simulink model "gm_sampleModel61753_pp_45_1_sub"  (R2023b)
settings: Solver=VariableStepAuto  StartTime=0.0  StopTime=10.0  RelTol=1e-3
libraries: simulink x43
(part 1 of 2)
settings Model: Creator=CW  LastModifiedBy=CW
settings OptimizationCC: BlockReduction=off  ConditionallyExecuteInputs=off
settings DebuggingCC: ArtificialAlgebraicLoopMsg=none  InheritedTsInSrcMsg=none

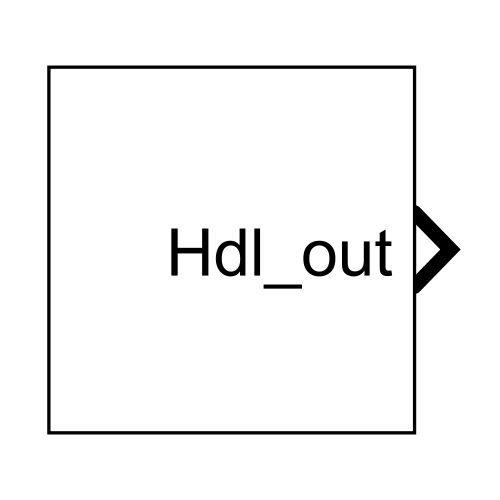
[thumbnail: Simulink's stored preview of the top-level diagram]
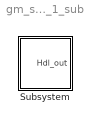
== system gm_sampleModel61753_pp_45_1_sub ==
  Subsystem : Subsystem

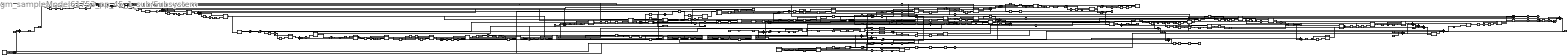
== system gm_sampleModel61753_pp_45_1_sub/Subsystem ==
  Reshape{,1..5} (6 alike) : Reshape
  cfblk1 : Subsystem
  cfblk{10,42,68,116,142,152} (6 alike) : Sum  OutDataTypeStr=uint8  AccumDataTypeStr=uint8  RndMeth=Nearest  SampleTime=1
  cfblk100 : Subsystem  mask(Real World Value Increment){}
      mask help: Simulink:masks:RealWorldValueIncrement_MD
      mask Display: disp('V++')
  cfblk101 : Subsystem
  cfblk{8,16,27,72,94,102,119..120,144,151} (10 alike) : Sum  Inputs=+  OutDataTypeStr=uint8
  cfblk{12,17,40,52,66,73,85,89,103,115,126} (11 alike) : Abs  SampleTime=1  OutDataTypeStr=uint8  SaturateOnIntegerOverflow=off
  cfblk{5,13,29,32,49,59,70,77,80..82,87,90,104,108,114,123,132,145} (19 alike) : Sum  OutDataTypeStr=uint8  AccumDataTypeStr=uint8  SampleTime=1
  cfblk{25..26,38,53,55,84,91,105,107} (9 alike) : MinMax  OutDataTypeStr=uint8
  cfblk{35,67,71,98,106,117} (6 alike) : Gain  Gain="fi(0,0,8,7,\"hex\",\"80\")"  ParamDataTypeStr=fixdt(0, 8, 7)  OutDataTypeStr=uint8  SampleTime=1
  cfblk109 : Subsystem
  cfblk10_const_val : Constant  Value=0  VectorParams1D=off  OutDataTypeStr=uint8  SampleTime=1
  cfblk{11,14,18,22,47,60,75,92,96,128,135} (11 alike) : Sum  Inputs=+-  OutDataTypeStr=uint8  AccumDataTypeStr=uint8  SampleTime=1
  cfblk{45,56,86,110,137,146..147} (7 alike) : Signum  SampleTime=1
  cfblk112 : Subsystem
  cfblk113 : Subsystem
  cfblk116_const_val : Constant  Value=0  VectorParams1D=off  OutDataTypeStr=uint8  SampleTime=1
  cfblk{15,23,28,34,36,118} (6 alike) : ComplexToRealImag  SampleTime=1
  cfblk121_inst : Subsystem
  cfblk124 : Subsystem
  cfblk125 : Subsystem
  cfblk127 : Subsystem
  cfblk129 : Subsystem
  cfblk130 : Subsystem  mask(Real World Value Increment){}
      mask help: Simulink:masks:RealWorldValueIncrement_MD
      mask Display: disp('V++')
  cfblk{39,44,61,78..79,99,131,136,149} (9 alike) : Product  Inputs=*/  OutDataTypeStr=uint8  RndMeth=Zero  SaturateOnIntegerOverflow=on  SampleTime=1
  cfblk133 : Subsystem
  cfblk134 : Subsystem
  cfblk138_inst : Subsystem
  cfblk139 : Subsystem  mask(Real World Value Increment){}
      mask help: Simulink:masks:RealWorldValueIncrement_MD
      mask Display: disp('V++')
  cfblk142_const_val : Constant  Value=0  VectorParams1D=off  OutDataTypeStr=uint8  SampleTime=1
  cfblk143 : Subsystem
  cfblk148 : Subsystem
  cfblk150 : Subsystem
  cfblk152_const_val : Constant  Value=0  VectorParams1D=off  OutDataTypeStr=uint8  SampleTime=1
  cfblk153 : Subsystem
  cfblk156 : Constant  OutDataTypeStr=uint8  SampleTime=1
  cfblk157 : Constant  OutDataTypeStr=uint8  SampleTime=1
  cfblk158 : Subsystem
  cfblk159 : Subsystem
  cfblk160 : Subsystem
  cfblk{161..164,166,168..171,173..178} (15 alike) : Delay  DelayLength=double(2)  InitialCondition=0  SampleTime=1
  cfblk165 : Subsystem
  cfblk167 : Subsystem
  cfblk172 : Subsystem
  cfblk{179,181..191,193} (13 alike) : DataTypeConversion  OutDataTypeStr=fixdt(0,8,0)
  cfblk180 : Subsystem
  cfblk19 : Subsystem
  cfblk192 : Subsystem
  cfblk194 : Subsystem
  cfblk2 : Subsystem  mask(Detect Rise Positive){vinit=double(0), InputProcessing=Elements as channels (sample based), OutDataTypeStr=uint8}
      mask prompts: vinit "Simulink:masks:InitialCondition_MP"; InputProcessing "Simulink:masks:InputProcessing_MP"; OutDataTypeStr "Simulink:masks:OutputDataType_MP"
      mask help: Simulink:masks:DetectRisePositive_MD
      mask init:
      | InputProcessing = 'Elements as channels (sample based)';
      | OutDataTypeStr = 'uint8';
      | vinit = double(0);
      mask TypeOptions InputProcessing: Simulink:masks:ColumnsAsChannelsFrameBased | Simulink:masks:ElementsAsChannelsSampleBased
      mask TypeOptions OutDataTypeStr: Simulink:masks:uint8 | Simulink:masks:boolean
      mask Display: fprintf('U > 0\n&  NOT\nU/z > 0')
  cfblk20 : Subsystem  mask(Real World Value Increment){}
      mask help: Simulink:masks:RealWorldValueIncrement_MD
      mask Display: disp('V++')
  cfblk21 : Subsystem
  cfblk24 : Subsystem
  cfblk28_term1 : Terminator
  cfblk3 : Subsystem  mask(Detect Rise Nonnegative){vinit=double(0), InputProcessing=Elements as channels (sample based), OutDataTypeStr=uint8}
      mask prompts: vinit "Simulink:masks:InitialCondition_MP"; InputProcessing "Simulink:masks:InputProcessing_MP"; OutDataTypeStr "Simulink:masks:OutputDataType_MP"
      mask help: Simulink:masks:DetectRiseNonnegative_MD
      mask init:
      | InputProcessing = 'Elements as channels (sample based)';
      | OutDataTypeStr = 'uint8';
      | vinit = double(0);
      mask TypeOptions InputProcessing: Simulink:masks:ColumnsAsChannelsFrameBased | Simulink:masks:ElementsAsChannelsSampleBased
      mask TypeOptions OutDataTypeStr: Simulink:masks:uint8 | Simulink:masks:boolean
      mask Display: fprintf('U >= 0\n&  NOT\nU/z >= 0')
  cfblk30 : Subsystem
  cfblk31_inst : Subsystem
  cfblk33 : Subsystem  mask(Real World Value Increment){}
      mask help: Simulink:masks:RealWorldValueIncrement_MD
      mask Display: disp('V++')
  cfblk37_inst : Subsystem
  cfblk4 : Subsystem  mask(Detect Fall Nonpositive){vinit=double(0), InputProcessing=Elements as channels (sample based), OutDataTypeStr=uint8}
      mask prompts: vinit "Simulink:masks:InitialCondition_MP"; InputProcessing "Simulink:masks:InputProcessing_MP"; OutDataTypeStr "Simulink:masks:OutputDataType_MP"
      mask help: Simulink:masks:DetectFallNonpositive_MD
      mask init:
      | InputProcessing = 'Elements as channels (sample based)';
      | OutDataTypeStr = 'uint8';
      | vinit = double(0);
      mask TypeOptions InputProcessing: Simulink:masks:ColumnsAsChannelsFrameBased | Simulink:masks:ElementsAsChannelsSampleBased
      mask TypeOptions OutDataTypeStr: Simulink:masks:uint8 | Simulink:masks:boolean
      mask Display: fprintf('U <= 0\n&  NOT\nU/z <= 0')
  cfblk41 : Subsystem
  cfblk42_const_val : Constant  Value=0  VectorParams1D=off  OutDataTypeStr=uint8  SampleTime=1
  cfblk43 : Subsystem
  cfblk46 : Subsystem
  cfblk48 : Subsystem
  cfblk50 : Subsystem
  cfblk51 : Subsystem
  cfblk54 : Subsystem
  cfblk57 : Subsystem
  cfblk58 : Subsystem
  cfblk62_inst : Subsystem
  cfblk65_inst : Subsystem
  cfblk68_const_val : Constant  Value=0  VectorParams1D=off  OutDataTypeStr=uint8  SampleTime=1
  cfblk69 : Subsystem
  cfblk6_inst : Subsystem
  cfblk7 : Subsystem
  cfblk74_inst : Subsystem
  cfblk76 : Subsystem
  cfblk83_inst : Subsystem
  cfblk88 : Subsystem
  cfblk9 : Subsystem
  cfblk93 : Subsystem
  cfblk95 : Subsystem
  cfblk97 : Subsystem
  compare{,1..2,4,6,11,14..16,20,22,24,26..28,33,36..38,41} (20 alike) : simulink/Logic and Bit Operations/Compare To Constant  relop=>=  const=0  OutDataTypeStr=boolean
  compare{5,7..10,12..13,17,19,21,23,25,29..30,32,34,39..40,42} (19 alike) : simulink/Logic and Bit Operations/Compare To Constant  relop=>=  const=255  OutDataTypeStr=boolean
  compare{3,18,31,35} (4 alike) : simulink/Logic and Bit Operations/Compare To Constant  relop=>=  const=1  OutDataTypeStr=boolean
  emi_{6,14,22,30,38,47,55,63,71,80,88,97,105,113,121,129,137,145,153,161,169,177,185,193,201,209,217,225,233,241,249,257,265,273,281,289,298,306,314,323,331,339,347} (43 alike) : DataTypeConversion  OutDataTypeStr=fixdt(0,8,0)
  emi_{7,15,23,31,56,64,89,106,114,122,146,186,210,218,250,266,282,299,307,348} (20 alike) : Delay  DelayLength=double(2)  InitialCondition=0  SampleTime=1
  emi_{48,130,234,332} (4 alike) : Delay  DelayLength=double(2)  InitialCondition=1  SampleTime=1
  emi_{39,72,81,98,138,154,162,170,178,194,202,226,242,258,274,290,315,324,340} (19 alike) : Delay  DelayLength=double(2)  InitialCondition=255  SampleTime=1
  Hdl_out : Outport  OutDataTypeStr=uint8  SampleTime=1
  wires:
  cfblk1/1(emi_2) -> cfblk60/1
  cfblk10/1 -> cfblk104/1
  cfblk100/1(y) -> cfblk189/1
  cfblk101/1(emi_18) -> cfblk25/1
  cfblk102/1 -> cfblk44/1, cfblk79/2
  cfblk103/1 -> cfblk147/1, cfblk100/1(u)
  cfblk104/1 -> cfblk176/1
  cfblk105/1 -> emi_130/1, cfblk148/1(emi_124), cfblk149/1
  cfblk106/1 -> cfblk47/2, cfblk146/1
  cfblk107/1 -> cfblk77/2, cfblk14/1
  cfblk108/1 -> emi_266/1, cfblk48/1(emi_260), cfblk27/1
  cfblk109/1(emi_26) -> cfblk151/1
  cfblk11/1 -> cfblk80/2
  cfblk110/1 -> emi_218/1, cfblk24/1(emi_212), cfblk61/2
  Reshape/1 -> cfblk85/1, emi_48/1, cfblk113/1(emi_41)
  cfblk112/1(emi_34) -> cfblk81/2
  cfblk113/1(emi_42) -> cfblk44/2
  cfblk113/2(emi_43) -> cfblk28/1
  cfblk114/1 -> cfblk12/1, emi_15/1, cfblk50/1(emi_9)
  cfblk115/1 -> emi_202/1, cfblk69/1(emi_196)
  cfblk116/1 -> cfblk22/2
  cfblk117/1 -> cfblk114/2
  cfblk118/1 -> cfblk10/1
  cfblk118/2 -> cfblk39/2
  cfblk119/1 -> emi_242/1, cfblk41/1(emi_236)
  cfblk12/1 -> cfblk29/2
  cfblk120/1 -> cfblk171/1
  cfblk121_inst/1(out1) -> cfblk56/1
  Reshape1/1 -> emi_56/1, cfblk51/1(emi_50)
  cfblk123/1 -> cfblk82/2
  cfblk124/1(emi_75) -> cfblk38/1
  cfblk124/2(emi_76) -> cfblk32/1
  cfblk125/1(emi_221) -> emi_98/1, cfblk133/1(emi_91)
  cfblk126/1 -> cfblk6_inst/1(in1)
  cfblk127/1(emi_173) -> cfblk75/1, cfblk32/2, cfblk61/1
  cfblk128/1 -> emi_138/1, cfblk150/1(emi_132)
  cfblk129/1(emi_84) -> cfblk22/1
  cfblk13/1 -> emi_31/1, cfblk109/1(emi_25)
  cfblk130/1(y) -> cfblk182/1
  cfblk131/1 -> cfblk128/1
  cfblk132/1 -> cfblk183/1
  cfblk133/1(emi_92) -> cfblk131/1
  cfblk133/2(emi_93) -> cfblk96/1
  cfblk134/1(emi_101) -> emi_114/1, cfblk143/1(emi_108)
  cfblk135/1 -> cfblk71/1
  cfblk136/1 -> cfblk72/1
  cfblk137/1 -> cfblk17/1
  cfblk138_inst/1(out1) -> cfblk102/1
  cfblk139/1(y) -> cfblk65_inst/2(in2), cfblk158/1(In1)
  cfblk14/1 -> emi_194/1, cfblk194/1(emi_188)
  Reshape2/1 -> cfblk45/1
  Reshape3/1 -> cfblk126/1
  cfblk142/1 -> cfblk92/1
  cfblk143/1(emi_109) -> cfblk163/1
  cfblk144/1 -> cfblk59/1, emi_340/1, cfblk95/1(emi_334)
  cfblk145/1 -> cfblk47/1
  cfblk146/1 -> cfblk3/1(U)
  cfblk147/1 -> cfblk136/1
  cfblk148/1(emi_125) -> cfblk145/1
  cfblk149/1 -> cfblk92/2
  cfblk15/1 -> Reshape3/1
  cfblk15/2 -> cfblk79/1
  cfblk150/1(emi_133) -> cfblk65_inst/1(in1), cfblk132/2, cfblk121_inst/2(in2)
  cfblk151/1 -> cfblk18/2
  cfblk152/1 -> emi_226/1, cfblk125/1(emi_220)
  cfblk153/1(emi_141) -> cfblk5/2
  cfblk156/1 -> cfblk35/1
  cfblk157/1 -> cfblk116/1
  cfblk158/1(Out1) -> cfblk138_inst/1(in1)
  cfblk159/1(emi_157) -> cfblk152/1, cfblk144/1
  cfblk16/1 -> cfblk42/1
  cfblk160/1(Out1) -> cfblk132/1, cfblk110/1
  cfblk161/1 -> emi_7/1, cfblk1/1(emi_1)
  cfblk162/1 -> cfblk114/1
  cfblk163/1 -> cfblk5/1
  cfblk164/1 -> cfblk60/2
  cfblk165/1(emi_117) -> cfblk18/1
  cfblk166/1 -> cfblk131/2
  cfblk167/1(emi_59) -> cfblk145/2
  cfblk168/1 -> cfblk78/2
  cfblk169/1 -> cfblk37_inst/1(in1)
  cfblk17/1 -> cfblk123/1
  cfblk170/1 -> cfblk11/1
  cfblk171/1 -> cfblk99/2
  cfblk172/1(emi_67) -> cfblk136/2
  cfblk173/1 -> cfblk80/1
  cfblk174/1 -> cfblk31_inst/1(in1)
  cfblk175/1 -> cfblk13/1
  cfblk176/1 -> cfblk29/1
  cfblk177/1 -> cfblk70/2
  cfblk178/1 -> emi_210/1, cfblk21/1(emi_204)
  cfblk179/1 -> cfblk135/1, cfblk166/1
  cfblk18/1 -> emi_348/1, cfblk97/1(emi_342)
  cfblk180/1(emi_149) -> cfblk74_inst/1(in1)
  cfblk181/1 -> cfblk74_inst/2(in2)
  cfblk182/1 -> emi_332/1, cfblk93/1(emi_326)
  cfblk183/1 -> cfblk130/1(u)
  cfblk184/1 -> emi_122/1, cfblk165/1(emi_116)
  cfblk185/1 -> cfblk31_inst/2(in2), cfblk181/1
  cfblk186/1 -> emi_299/1, cfblk7/1(emi_292)
  cfblk187/1 -> Reshape/1
  cfblk188/1 -> Reshape4/1, cfblk121_inst/1(in1)
  cfblk189/1 -> cfblk34/1
  cfblk19/1(emi_165) -> cfblk87/1
  cfblk190/1 -> cfblk193/1
  cfblk191/1 -> emi_234/1, cfblk30/1(emi_228)
  cfblk192/1(emi_181) -> emi_89/1, cfblk129/1(emi_83)
  cfblk193/1 -> cfblk83_inst/1(in1)
  cfblk194/1(emi_189) -> cfblk83_inst/2(in2)
  cfblk2/1(Y) -> cfblk14/2, cfblk177/1
  cfblk20/1(y) -> cfblk173/1
  cfblk21/1(emi_205) -> emi_282/1, cfblk57/1(emi_276), cfblk149/2
  cfblk22/1 -> cfblk142/1
  cfblk23/1 -> cfblk62_inst/1(in1)
  cfblk23/2 -> cfblk160/1(In1)
  cfblk24/1(emi_213) -> cfblk178/1
  cfblk25/1 -> cfblk36/1
  cfblk26/1 -> cfblk6_inst/2(in2)
  cfblk27/1 -> cfblk90/1
  cfblk28/1 -> Reshape1/1
  cfblk28/2 -> cfblk28_term1/1
  cfblk29/1 -> emi_146/1, cfblk153/1(emi_140)
  cfblk3/1(Y) -> cfblk49/1, cfblk117/1
  cfblk30/1(emi_229) -> cfblk190/1
  cfblk31_inst/1(out1) -> cfblk70/1
  cfblk32/1 -> cfblk86/1
  cfblk33/1(y) -> cfblk170/1
  cfblk34/1 -> cfblk187/1
  cfblk34/2 -> cfblk188/1
  cfblk35/1 -> cfblk52/1
  cfblk36/1 -> cfblk8/1
  cfblk36/2 -> cfblk15/1
  cfblk37_inst/1(out1) -> emi_315/1, cfblk88/1(emi_309)
  cfblk38/1 -> cfblk84/1
  cfblk39/1 -> cfblk4/1(U)
  cfblk4/1(Y) -> cfblk186/1
  cfblk40/1 -> cfblk2/1(U)
  cfblk41/1(emi_237) -> cfblk77/1
  cfblk42/1 -> cfblk120/1
  cfblk43/1(emi_245) -> cfblk39/1
  cfblk44/1 -> cfblk169/1
  cfblk45/1 -> cfblk118/1
  cfblk46/1(emi_253) -> emi_39/1, cfblk112/1(emi_33)
  cfblk47/1 -> emi_250/1, cfblk43/1(emi_244), cfblk55/1
  cfblk48/1(emi_261) -> cfblk53/1
  cfblk49/1 -> cfblk161/1
  cfblk5/1 -> cfblk11/2
  cfblk50/1(emi_10) -> cfblk128/2
  cfblk51/1(emi_51) -> emi_307/1, cfblk76/1(emi_301)
  cfblk52/1 -> cfblk81/1
  cfblk53/1 -> cfblk105/1
  cfblk54/1(emi_269) -> cfblk78/1
  cfblk55/1 -> cfblk164/1
  cfblk56/1 -> cfblk99/1, cfblk119/1
  cfblk57/1(emi_277) -> cfblk23/1
  cfblk58/1(emi_285) -> cfblk20/1(u)
  cfblk59/1 -> cfblk26/1
  cfblk6_inst/1(out1) -> emi_81/1, cfblk124/1(emi_74)
  cfblk60/1 -> cfblk68/1
  cfblk61/1 -> emi_324/1, cfblk9/1(emi_317)
  cfblk62_inst/1(out1) -> cfblk59/2
  Reshape4/1 -> cfblk49/2
  Reshape5/1 -> cfblk13/2
  cfblk65_inst/1(out1) -> emi_154/1, cfblk180/1(emi_148)
  cfblk66/1 -> cfblk82/1, cfblk137/1
  cfblk67/1 -> cfblk162/1
  cfblk68/1 -> cfblk94/1
  cfblk69/1(emi_197) -> emi_178/1, cfblk127/1(emi_172)
  cfblk7/1(emi_293) -> cfblk184/1
  cfblk7/2(emi_294) -> cfblk185/1
  cfblk70/1 -> cfblk103/1
  cfblk71/1 -> emi_64/1, cfblk167/1(emi_58)
  cfblk72/1 -> emi_274/1, cfblk54/1(emi_268)
  cfblk73/1 -> cfblk37_inst/2(in2)
  cfblk74_inst/1(out1) -> cfblk179/1
  cfblk75/1 -> cfblk107/1
  cfblk76/1(emi_302) -> cfblk40/1
  cfblk77/1 -> cfblk89/1
  cfblk78/1 -> emi_162/1, cfblk159/1(emi_156)
  cfblk79/1 -> cfblk33/1(u)
  cfblk8/1 -> cfblk108/1
  cfblk80/1 -> cfblk90/2, cfblk135/2, cfblk108/2, cfblk98/1
  cfblk81/1 -> cfblk115/1
  cfblk82/1 -> cfblk96/2, cfblk168/1
  cfblk83_inst/1(out1) -> emi_186/1, cfblk192/1(emi_180)
  cfblk84/1 -> cfblk66/1
  cfblk85/1 -> cfblk191/1
  cfblk86/1 -> cfblk175/1
  cfblk87/1 -> cfblk123/2, emi_72/1, cfblk172/1(emi_66)
  cfblk88/1(emi_310) -> cfblk91/1
  cfblk89/1 -> cfblk138_inst/2(in2)
  cfblk9/1(emi_318) -> cfblk104/2
  cfblk9/2(emi_319) -> cfblk87/2
  cfblk90/1 -> emi_106/1, cfblk67/1, cfblk134/1(emi_100)
  cfblk91/1 -> emi_170/1, cfblk19/1(emi_164)
  cfblk92/1 -> cfblk62_inst/2(in2)
  cfblk93/1(emi_327) -> cfblk174/1
  cfblk94/1 -> Reshape5/1
  cfblk95/1(emi_335) -> cfblk75/2, emi_258/1, cfblk46/1(emi_252)
  cfblk96/1 -> cfblk139/1(u), cfblk16/1
  cfblk97/1(emi_343) -> Reshape2/1, cfblk106/1
  cfblk98/1 -> emi_23/1, cfblk101/1(emi_17)
  cfblk99/1 -> cfblk73/1, emi_290/1, cfblk58/1(emi_284)
  emi_105/1 -> compare/1
  emi_106/1 -> emi_105/1
  emi_113/1 -> compare1/1
  emi_114/1 -> emi_113/1
  emi_121/1 -> compare2/1
  emi_122/1 -> emi_121/1
  emi_129/1 -> compare3/1
  emi_130/1 -> emi_129/1
  emi_137/1 -> compare5/1
  emi_138/1 -> emi_137/1
  emi_14/1 -> compare4/1
  emi_145/1 -> compare6/1
  emi_146/1 -> emi_145/1
  emi_15/1 -> emi_14/1
  emi_153/1 -> compare7/1
  emi_154/1 -> emi_153/1
  emi_161/1 -> compare8/1
  emi_162/1 -> emi_161/1
  emi_169/1 -> compare9/1
  emi_170/1 -> emi_169/1
  emi_177/1 -> compare10/1
  emi_178/1 -> emi_177/1
  emi_185/1 -> compare11/1
  emi_186/1 -> emi_185/1
  emi_193/1 -> compare12/1
  emi_194/1 -> emi_193/1
  emi_201/1 -> compare13/1
  emi_202/1 -> emi_201/1
  emi_209/1 -> compare14/1
  emi_210/1 -> emi_209/1
  emi_217/1 -> compare16/1
  emi_218/1 -> emi_217/1
  emi_22/1 -> compare15/1
  emi_225/1 -> compare17/1
  emi_226/1 -> emi_225/1
  emi_23/1 -> emi_22/1
  emi_233/1 -> compare18/1
  emi_234/1 -> emi_233/1
  emi_241/1 -> compare19/1
  emi_242/1 -> emi_241/1
  emi_249/1 -> compare20/1
  emi_250/1 -> emi_249/1
  emi_257/1 -> compare21/1
  emi_258/1 -> emi_257/1
  emi_265/1 -> compare22/1
  emi_266/1 -> emi_265/1
  emi_273/1 -> compare23/1
  emi_274/1 -> emi_273/1
  emi_281/1 -> compare24/1
  emi_282/1 -> emi_281/1
  emi_289/1 -> compare25/1
  emi_290/1 -> emi_289/1
  emi_298/1 -> compare27/1
  emi_299/1 -> emi_298/1
  emi_30/1 -> compare26/1
  emi_306/1 -> compare28/1
  emi_307/1 -> emi_306/1
  emi_31/1 -> emi_30/1
  emi_314/1 -> compare29/1
  emi_315/1 -> emi_314/1
  emi_323/1 -> compare30/1
  emi_324/1 -> emi_323/1
  emi_331/1 -> compare31/1
  emi_332/1 -> emi_331/1
  emi_339/1 -> compare32/1
  emi_340/1 -> emi_339/1
  emi_347/1 -> compare33/1
  emi_348/1 -> emi_347/1
  emi_38/1 -> compare34/1
  emi_39/1 -> emi_38/1
  emi_47/1 -> compare35/1
  emi_48/1 -> emi_47/1
  emi_55/1 -> compare37/1
  emi_56/1 -> emi_55/1
  emi_6/1 -> compare36/1
  emi_63/1 -> compare38/1
  emi_64/1 -> emi_63/1, Hdl_out/1
  emi_7/1 -> emi_6/1
  emi_71/1 -> compare39/1
  emi_72/1 -> emi_71/1
  emi_80/1 -> compare40/1
  emi_81/1 -> emi_80/1
  emi_88/1 -> compare41/1
  emi_89/1 -> emi_88/1
  emi_97/1 -> compare42/1
  emi_98/1 -> emi_97/1
  cfblk10_const_val/1 -> cfblk10/2
  cfblk116_const_val/1 -> cfblk116/2
  cfblk142_const_val/1 -> cfblk142/2
  cfblk152_const_val/1 -> cfblk152/2
  cfblk42_const_val/1 -> cfblk42/2
  cfblk68_const_val/1 -> cfblk68/2
  compare/1 -> cfblk134/2(Action Port)
  compare1/1 -> cfblk143/2(Action Port)
  compare2/1 -> cfblk165/2(Action Port)
  compare3/1 -> cfblk148/2(Action Port)
  compare4/1 -> cfblk50/2(Action Port)
  compare5/1 -> cfblk150/2(Action Port)
  compare6/1 -> cfblk153/2(Action Port)
  compare7/1 -> cfblk180/2(Action Port)
  compare8/1 -> cfblk159/2(Action Port)
  compare9/1 -> cfblk19/2(Action Port)
  compare10/1 -> cfblk127/2(Action Port)
  compare11/1 -> cfblk192/2(Action Port)
  compare12/1 -> cfblk194/2(Action Port)
  compare13/1 -> cfblk69/2(Action Port)
  compare14/1 -> cfblk21/2(Action Port)
  compare15/1 -> cfblk101/2(Action Port)
  compare16/1 -> cfblk24/2(Action Port)
  compare17/1 -> cfblk125/2(Action Port)
  compare18/1 -> cfblk30/2(Action Port)
  compare19/1 -> cfblk41/2(Action Port)
  compare20/1 -> cfblk43/2(Action Port)
  compare21/1 -> cfblk46/2(Action Port)
  compare22/1 -> cfblk48/2(Action Port)
  compare23/1 -> cfblk54/2(Action Port)
  compare24/1 -> cfblk57/2(Action Port)
  compare25/1 -> cfblk58/2(Action Port)
  compare26/1 -> cfblk109/2(Action Port)
  compare27/1 -> cfblk7/2(Action Port)
  compare28/1 -> cfblk76/2(Action Port)
  compare29/1 -> cfblk88/2(Action Port)
  compare30/1 -> cfblk9/2(Action Port)
  compare31/1 -> cfblk93/2(Action Port)
  compare32/1 -> cfblk95/2(Action Port)
  compare33/1 -> cfblk97/2(Action Port)
  compare34/1 -> cfblk112/2(Action Port)
  compare35/1 -> cfblk113/2(Action Port)
  compare36/1 -> cfblk1/2(Action Port)
  compare37/1 -> cfblk51/2(Action Port)
  compare38/1 -> cfblk167/2(Action Port)
  compare39/1 -> cfblk172/2(Action Port)
  compare40/1 -> cfblk124/2(Action Port)
  compare41/1 -> cfblk129/2(Action Port)
  compare42/1 -> cfblk133/2(Action Port)

== system gm_sampleModel61753_pp_45_1_sub/Subsystem/cfblk1 ==
  emi_1 : Inport  OutDataTypeStr=uint8  PortDimensions=1  SampleTime=1
  Action Port : Inport  Port=2  OutDataTypeStr=boolean  SampleTime=1
  cfblk1 : Subsystem  mask(Detect Rise Nonnegative){vinit=double(0), InputProcessing=Elements as channels (sample based), OutDataTypeStr=uint8}
      mask prompts: vinit "Simulink:masks:InitialCondition_MP"; InputProcessing "Simulink:masks:InputProcessing_MP"; OutDataTypeStr "Simulink:masks:OutputDataType_MP"
      mask help: Simulink:masks:DetectRiseNonnegative_MD
      mask TypeOptions InputProcessing: Simulink:masks:ColumnsAsChannelsFrameBased | Simulink:masks:ElementsAsChannelsSampleBased
      mask TypeOptions OutDataTypeStr: Simulink:masks:uint8 | Simulink:masks:boolean
      mask Display: fprintf('U >= 0\n&  NOT\nU/z >= 0')
  cfblk1_out1bypassMux : MultiPortSwitch  DataPortOrder=Zero-based contiguous  Inputs=2  zeroidx=on  OutDataTypeStr=uint8  SampleTime=1  SaturateOnIntegerOverflow=off  InputSameDT=off
  emi_2_bypass : UnitDelay  InitialCondition="fi(0,0,8,0,\"hex\",\"00\")"  SampleTime=1
  emi_2 : Outport  SampleTime=1  InitialOutput=0
  wires:
  Action Port/1 -> cfblk1_out1bypassMux/1, cfblk1/2(Action Port_out2)
  emi_1/1 -> cfblk1/1(U)
  cfblk1/1(Y) -> cfblk1_out1bypassMux/3
  cfblk1_out1bypassMux/1 -> emi_2_bypass/1, emi_2/1
  emi_2_bypass/1 -> cfblk1_out1bypassMux/2

== system gm_sampleModel61753_pp_45_1_sub/Subsystem/cfblk100 ==
  u : Inport  OutDataTypeStr=uint8  SampleTime=1
  FixPt Constant : Constant  DisableCoverage=on  OutDataTypeStr=Inherit: Inherit via back propagation  SampleTime=-1
  FixPt Data Type Duplicate : DataTypeDuplicate  DisableCoverage=on  NumInputPorts=3
  FixPt Sum1 : Sum  OutDataTypeStr=Inherit: Inherit via back propagation  InputSameDT=on  LockScale=on
  y : Outport  SampleTime=1
  wires:
  u/1 -> FixPt Sum1/1, FixPt Data Type Duplicate/2
  FixPt Constant/1 -> FixPt Sum1/2, FixPt Data Type Duplicate/3
  FixPt Sum1/1 -> FixPt Data Type Duplicate/1, y/1

== system gm_sampleModel61753_pp_45_1_sub/Subsystem/cfblk101 ==
  emi_17 : Inport  OutDataTypeStr=uint8  PortDimensions=1  SampleTime=1
  Action Port : Inport  Port=2  OutDataTypeStr=boolean  SampleTime=1
  cfblk101 : Abs  SampleTime=1  OutDataTypeStr=uint8  SaturateOnIntegerOverflow=off
  cfblk101_out1bypassMux : MultiPortSwitch  DataPortOrder=Zero-based contiguous  Inputs=2  zeroidx=on  OutDataTypeStr=uint8  SampleTime=1  SaturateOnIntegerOverflow=off  InputSameDT=off
  emi_18_bypass : UnitDelay  InitialCondition="fi(0,0,8,0,\"hex\",\"00\")"  SampleTime=1
  emi_18 : Outport  SampleTime=1  InitialOutput=0
  wires:
  Action Port/1 -> cfblk101_out1bypassMux/1
  emi_17/1 -> cfblk101/1
  cfblk101/1 -> cfblk101_out1bypassMux/3
  cfblk101_out1bypassMux/1 -> emi_18_bypass/1, emi_18/1
  emi_18_bypass/1 -> cfblk101_out1bypassMux/2

== system gm_sampleModel61753_pp_45_1_sub/Subsystem/cfblk109 ==
  emi_25 : Inport  OutDataTypeStr=uint8  PortDimensions=1  SampleTime=1
  Action Port : Inport  Port=2  OutDataTypeStr=boolean  SampleTime=1
  cfblk109 : Abs  SampleTime=1  OutDataTypeStr=uint8  SaturateOnIntegerOverflow=off
  cfblk109_out1bypassMux : MultiPortSwitch  DataPortOrder=Zero-based contiguous  Inputs=2  zeroidx=on  OutDataTypeStr=uint8  SampleTime=1  SaturateOnIntegerOverflow=off  InputSameDT=off
  emi_26_bypass : UnitDelay  InitialCondition="fi(0,0,8,0,\"hex\",\"00\")"  SampleTime=1
  emi_26 : Outport  SampleTime=1  InitialOutput=0
  wires:
  Action Port/1 -> cfblk109_out1bypassMux/1
  emi_25/1 -> cfblk109/1
  cfblk109/1 -> cfblk109_out1bypassMux/3
  cfblk109_out1bypassMux/1 -> emi_26_bypass/1, emi_26/1
  emi_26_bypass/1 -> cfblk109_out1bypassMux/2

== system gm_sampleModel61753_pp_45_1_sub/Subsystem/cfblk112 ==
  emi_33 : Inport  OutDataTypeStr=uint8  PortDimensions=1  SampleTime=1
  Action Port : Inport  Port=2  OutDataTypeStr=boolean  SampleTime=1
  cfblk112 : Sum  Inputs=+
  cfblk112_out1bypassMux : MultiPortSwitch  DataPortOrder=Zero-based contiguous  Inputs=2  zeroidx=on  OutDataTypeStr=uint8  SampleTime=1  SaturateOnIntegerOverflow=off  InputSameDT=off
  emi_34_bypass : UnitDelay  InitialCondition="fi(0,0,8,0,\"hex\",\"00\")"  SampleTime=1
  emi_34 : Outport  SampleTime=1  InitialOutput=0
  wires:
  Action Port/1 -> cfblk112_out1bypassMux/1
  emi_33/1 -> cfblk112/1
  cfblk112/1 -> cfblk112_out1bypassMux/3
  cfblk112_out1bypassMux/1 -> emi_34_bypass/1, emi_34/1
  emi_34_bypass/1 -> cfblk112_out1bypassMux/2

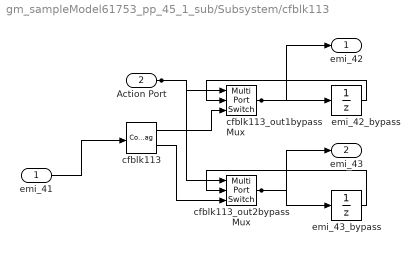
== system gm_sampleModel61753_pp_45_1_sub/Subsystem/cfblk113 ==
  emi_41 : Inport  OutDataTypeStr=uint8  PortDimensions=1  SampleTime=1
  Action Port : Inport  Port=2  OutDataTypeStr=boolean  SampleTime=1
  cfblk113 : ComplexToRealImag  SampleTime=1
  cfblk113_out1bypassMux : MultiPortSwitch  DataPortOrder=Zero-based contiguous  Inputs=2  zeroidx=on  OutDataTypeStr=uint8  SampleTime=1  SaturateOnIntegerOverflow=off  InputSameDT=off
  cfblk113_out2bypassMux : MultiPortSwitch  DataPortOrder=Zero-based contiguous  Inputs=2  zeroidx=on  OutDataTypeStr=uint8  SampleTime=1  SaturateOnIntegerOverflow=off  InputSameDT=off
  emi_42_bypass : UnitDelay  InitialCondition="fi(0,0,8,0,\"hex\",\"00\")"  SampleTime=1
  emi_43_bypass : UnitDelay  InitialCondition="fi(0,0,8,0,\"hex\",\"00\")"  SampleTime=1
  emi_42 : Outport  SampleTime=1  InitialOutput=0
  emi_43 : Outport  Port=2  SampleTime=1  InitialOutput=0
  wires:
  Action Port/1 -> cfblk113_out2bypassMux/1, cfblk113_out1bypassMux/1
  emi_41/1 -> cfblk113/1
  cfblk113/1 -> cfblk113_out1bypassMux/3
  cfblk113/2 -> cfblk113_out2bypassMux/3
  cfblk113_out1bypassMux/1 -> emi_42_bypass/1, emi_42/1
  emi_42_bypass/1 -> cfblk113_out1bypassMux/2
  cfblk113_out2bypassMux/1 -> emi_43_bypass/1, emi_43/1
  emi_43_bypass/1 -> cfblk113_out2bypassMux/2

== system gm_sampleModel61753_pp_45_1_sub/Subsystem/cfblk121_inst ==
  in1 : Inport  OutDataTypeStr=uint8  SampleTime=1
  in2 : Inport  Port=2  OutDataTypeStr=uint8  SampleTime=1
  mul_cfblk121_dotp_mulcomp : Product  Inputs=**  OutDataTypeStr=uint8  SampleTime=1
  out1 : Outport  OutDataTypeStr=uint8  SampleTime=1
  wires:
  in1/1 -> mul_cfblk121_dotp_mulcomp/1
  in2/1 -> mul_cfblk121_dotp_mulcomp/2
  mul_cfblk121_dotp_mulcomp/1 -> out1/1

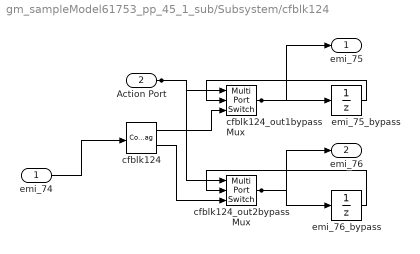
== system gm_sampleModel61753_pp_45_1_sub/Subsystem/cfblk124 ==
  emi_74 : Inport  OutDataTypeStr=uint8  PortDimensions=1  SampleTime=1
  Action Port : Inport  Port=2  OutDataTypeStr=boolean  SampleTime=1
  cfblk124 : ComplexToRealImag  SampleTime=1
  cfblk124_out1bypassMux : MultiPortSwitch  DataPortOrder=Zero-based contiguous  Inputs=2  zeroidx=on  OutDataTypeStr=uint8  SampleTime=1  SaturateOnIntegerOverflow=off  InputSameDT=off
  cfblk124_out2bypassMux : MultiPortSwitch  DataPortOrder=Zero-based contiguous  Inputs=2  zeroidx=on  OutDataTypeStr=uint8  SampleTime=1  SaturateOnIntegerOverflow=off  InputSameDT=off
  emi_75_bypass : UnitDelay  InitialCondition="fi(0,0,8,0,\"hex\",\"00\")"  SampleTime=1
  emi_76_bypass : UnitDelay  InitialCondition="fi(0,0,8,0,\"hex\",\"00\")"  SampleTime=1
  emi_75 : Outport  SampleTime=1  InitialOutput=0
  emi_76 : Outport  Port=2  SampleTime=1  InitialOutput=0
  wires:
  Action Port/1 -> cfblk124_out2bypassMux/1, cfblk124_out1bypassMux/1
  emi_74/1 -> cfblk124/1
  cfblk124/1 -> cfblk124_out1bypassMux/3
  cfblk124/2 -> cfblk124_out2bypassMux/3
  cfblk124_out1bypassMux/1 -> emi_75_bypass/1, emi_75/1
  emi_75_bypass/1 -> cfblk124_out1bypassMux/2
  cfblk124_out2bypassMux/1 -> emi_76_bypass/1, emi_76/1
  emi_76_bypass/1 -> cfblk124_out2bypassMux/2

== system gm_sampleModel61753_pp_45_1_sub/Subsystem/cfblk125 ==
  emi_220 : Inport  OutDataTypeStr=uint8  PortDimensions=1  SampleTime=1
  Action Port : Inport  Port=2  OutDataTypeStr=boolean  SampleTime=1
  cfblk125 : Sum  Inputs=+
  cfblk125_out1bypassMux : MultiPortSwitch  DataPortOrder=Zero-based contiguous  Inputs=2  zeroidx=on  OutDataTypeStr=uint8  SampleTime=1  SaturateOnIntegerOverflow=off  InputSameDT=off
  emi_221_bypass : UnitDelay  InitialCondition="fi(0,0,8,0,\"hex\",\"00\")"  SampleTime=1
  emi_221 : Outport  SampleTime=1  InitialOutput=0
  wires:
  Action Port/1 -> cfblk125_out1bypassMux/1
  emi_220/1 -> cfblk125/1
  cfblk125/1 -> cfblk125_out1bypassMux/3
  cfblk125_out1bypassMux/1 -> emi_221_bypass/1, emi_221/1
  emi_221_bypass/1 -> cfblk125_out1bypassMux/2

== system gm_sampleModel61753_pp_45_1_sub/Subsystem/cfblk127 ==
  emi_172 : Inport  OutDataTypeStr=uint8  PortDimensions=1  SampleTime=1
  Action Port : Inport  Port=2  OutDataTypeStr=boolean  SampleTime=1
  cfblk127 : Signum  SampleTime=1
  cfblk127_out1bypassMux : MultiPortSwitch  DataPortOrder=Zero-based contiguous  Inputs=2  zeroidx=on  OutDataTypeStr=uint8  SampleTime=1  SaturateOnIntegerOverflow=off  InputSameDT=off
  emi_173_bypass : UnitDelay  InitialCondition="fi(0,0,8,0,\"hex\",\"00\")"  SampleTime=1
  emi_173 : Outport  SampleTime=1  InitialOutput=0
  wires:
  Action Port/1 -> cfblk127_out1bypassMux/1
  emi_172/1 -> cfblk127/1
  cfblk127/1 -> cfblk127_out1bypassMux/3
  cfblk127_out1bypassMux/1 -> emi_173_bypass/1, emi_173/1
  emi_173_bypass/1 -> cfblk127_out1bypassMux/2

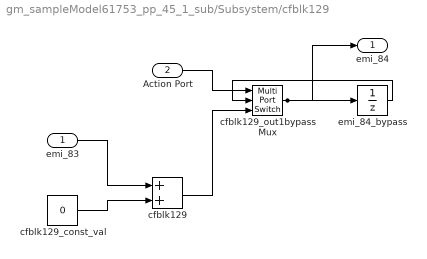
== system gm_sampleModel61753_pp_45_1_sub/Subsystem/cfblk129 ==
  emi_83 : Inport  OutDataTypeStr=uint8  PortDimensions=1  SampleTime=1
  Action Port : Inport  Port=2  OutDataTypeStr=boolean  SampleTime=1
  cfblk129 : Sum  OutDataTypeStr=uint8  AccumDataTypeStr=uint8  RndMeth=Nearest  SampleTime=1
  cfblk129_const_val : Constant  Value=0  VectorParams1D=off  OutDataTypeStr=uint8  SampleTime=1
  cfblk129_out1bypassMux : MultiPortSwitch  DataPortOrder=Zero-based contiguous  Inputs=2  zeroidx=on  OutDataTypeStr=uint8  SampleTime=1  SaturateOnIntegerOverflow=off  InputSameDT=off
  emi_84_bypass : UnitDelay  InitialCondition="fi(0,0,8,0,\"hex\",\"00\")"  SampleTime=1
  emi_84 : Outport  SampleTime=1  InitialOutput=0
  wires:
  Action Port/1 -> cfblk129_out1bypassMux/1
  emi_83/1 -> cfblk129/1
  cfblk129/1 -> cfblk129_out1bypassMux/3
  cfblk129_out1bypassMux/1 -> emi_84_bypass/1, emi_84/1
  emi_84_bypass/1 -> cfblk129_out1bypassMux/2
  cfblk129_const_val/1 -> cfblk129/2

== system gm_sampleModel61753_pp_45_1_sub/Subsystem/cfblk130 ==
  u : Inport  OutDataTypeStr=uint8  SampleTime=1
  FixPt Constant : Constant  DisableCoverage=on  OutDataTypeStr=Inherit: Inherit via back propagation  SampleTime=-1
  FixPt Data Type Duplicate : DataTypeDuplicate  DisableCoverage=on  NumInputPorts=3
  FixPt Sum1 : Sum  OutDataTypeStr=Inherit: Inherit via back propagation  InputSameDT=on  LockScale=on
  y : Outport  SampleTime=1
  wires:
  u/1 -> FixPt Sum1/1, FixPt Data Type Duplicate/2
  FixPt Constant/1 -> FixPt Sum1/2, FixPt Data Type Duplicate/3
  FixPt Sum1/1 -> FixPt Data Type Duplicate/1, y/1

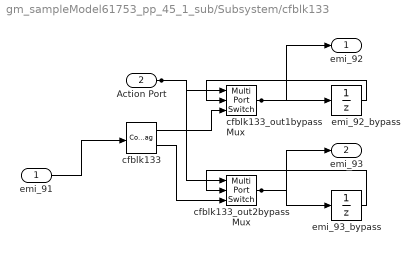
== system gm_sampleModel61753_pp_45_1_sub/Subsystem/cfblk133 ==
  emi_91 : Inport  OutDataTypeStr=uint8  PortDimensions=1  SampleTime=1
  Action Port : Inport  Port=2  OutDataTypeStr=boolean  SampleTime=1
  cfblk133 : ComplexToRealImag  SampleTime=1
  cfblk133_out1bypassMux : MultiPortSwitch  DataPortOrder=Zero-based contiguous  Inputs=2  zeroidx=on  OutDataTypeStr=uint8  SampleTime=1  SaturateOnIntegerOverflow=off  InputSameDT=off
  cfblk133_out2bypassMux : MultiPortSwitch  DataPortOrder=Zero-based contiguous  Inputs=2  zeroidx=on  OutDataTypeStr=uint8  SampleTime=1  SaturateOnIntegerOverflow=off  InputSameDT=off
  emi_92_bypass : UnitDelay  InitialCondition="fi(0,0,8,0,\"hex\",\"00\")"  SampleTime=1
  emi_93_bypass : UnitDelay  InitialCondition="fi(0,0,8,0,\"hex\",\"00\")"  SampleTime=1
  emi_92 : Outport  SampleTime=1  InitialOutput=0
  emi_93 : Outport  Port=2  SampleTime=1  InitialOutput=0
  wires:
  Action Port/1 -> cfblk133_out2bypassMux/1, cfblk133_out1bypassMux/1
  emi_91/1 -> cfblk133/1
  cfblk133/1 -> cfblk133_out1bypassMux/3
  cfblk133/2 -> cfblk133_out2bypassMux/3
  cfblk133_out1bypassMux/1 -> emi_92_bypass/1, emi_92/1
  emi_92_bypass/1 -> cfblk133_out1bypassMux/2
  cfblk133_out2bypassMux/1 -> emi_93_bypass/1, emi_93/1
  emi_93_bypass/1 -> cfblk133_out2bypassMux/2

== system gm_sampleModel61753_pp_45_1_sub/Subsystem/cfblk134 ==
  emi_100 : Inport  OutDataTypeStr=uint8  PortDimensions=1  SampleTime=1
  Action Port : Inport  Port=2  OutDataTypeStr=boolean  SampleTime=1
  cfblk134 : Sum  Inputs=+
  cfblk134_out1bypassMux : MultiPortSwitch  DataPortOrder=Zero-based contiguous  Inputs=2  zeroidx=on  OutDataTypeStr=uint8  SampleTime=1  SaturateOnIntegerOverflow=off  InputSameDT=off
  emi_101_bypass : UnitDelay  InitialCondition="fi(0,0,8,0,\"hex\",\"00\")"  SampleTime=1
  emi_101 : Outport  SampleTime=1  InitialOutput=0
  wires:
  Action Port/1 -> cfblk134_out1bypassMux/1
  emi_100/1 -> cfblk134/1
  cfblk134/1 -> cfblk134_out1bypassMux/3
  cfblk134_out1bypassMux/1 -> emi_101_bypass/1, emi_101/1
  emi_101_bypass/1 -> cfblk134_out1bypassMux/2

== system gm_sampleModel61753_pp_45_1_sub/Subsystem/cfblk138_inst ==
  in1 : Inport  OutDataTypeStr=uint8  SampleTime=1
  in2 : Inport  Port=2  OutDataTypeStr=uint8  SampleTime=1
  mul_cfblk138_dotp_mulcomp : Product  Inputs=**  OutDataTypeStr=uint8  SampleTime=1
  out1 : Outport  OutDataTypeStr=uint8  SampleTime=1
  wires:
  in1/1 -> mul_cfblk138_dotp_mulcomp/1
  in2/1 -> mul_cfblk138_dotp_mulcomp/2
  mul_cfblk138_dotp_mulcomp/1 -> out1/1

== system gm_sampleModel61753_pp_45_1_sub/Subsystem/cfblk139 ==
  u : Inport  OutDataTypeStr=uint8  SampleTime=1
  FixPt Constant : Constant  DisableCoverage=on  OutDataTypeStr=Inherit: Inherit via back propagation  SampleTime=-1
  FixPt Data Type Duplicate : DataTypeDuplicate  DisableCoverage=on  NumInputPorts=3
  FixPt Sum1 : Sum  OutDataTypeStr=Inherit: Inherit via back propagation  InputSameDT=on  LockScale=on
  y : Outport  SampleTime=1
  wires:
  u/1 -> FixPt Sum1/1, FixPt Data Type Duplicate/2
  FixPt Constant/1 -> FixPt Sum1/2, FixPt Data Type Duplicate/3
  FixPt Sum1/1 -> FixPt Data Type Duplicate/1, y/1

== system gm_sampleModel61753_pp_45_1_sub/Subsystem/cfblk143 ==
  emi_108 : Inport  OutDataTypeStr=uint8  PortDimensions=1  SampleTime=1
  Action Port : Inport  Port=2  OutDataTypeStr=boolean  SampleTime=1
  cfblk143 : MinMax
  cfblk143_out1bypassMux : MultiPortSwitch  DataPortOrder=Zero-based contiguous  Inputs=2  zeroidx=on  OutDataTypeStr=uint8  SampleTime=1  SaturateOnIntegerOverflow=off  InputSameDT=off
  emi_109_bypass : UnitDelay  InitialCondition="fi(0,0,8,0,\"hex\",\"00\")"  SampleTime=1
  emi_109 : Outport  SampleTime=1  InitialOutput=0
  wires:
  Action Port/1 -> cfblk143_out1bypassMux/1
  emi_108/1 -> cfblk143/1
  cfblk143/1 -> cfblk143_out1bypassMux/3
  cfblk143_out1bypassMux/1 -> emi_109_bypass/1, emi_109/1
  emi_109_bypass/1 -> cfblk143_out1bypassMux/2

== system gm_sampleModel61753_pp_45_1_sub/Subsystem/cfblk148 ==
  emi_124 : Inport  OutDataTypeStr=uint8  PortDimensions=1  SampleTime=1
  Action Port : Inport  Port=2  OutDataTypeStr=boolean  SampleTime=1
  cfblk148 : Signum  SampleTime=1
  cfblk148_out1bypassMux : MultiPortSwitch  DataPortOrder=Zero-based contiguous  Inputs=2  zeroidx=on  OutDataTypeStr=uint8  SampleTime=1  SaturateOnIntegerOverflow=off  InputSameDT=off
  emi_125_bypass : UnitDelay  InitialCondition="fi(0,0,8,0,\"hex\",\"00\")"  SampleTime=1
  emi_125 : Outport  SampleTime=1  InitialOutput=0
  wires:
  Action Port/1 -> cfblk148_out1bypassMux/1
  emi_124/1 -> cfblk148/1
  cfblk148/1 -> cfblk148_out1bypassMux/3
  cfblk148_out1bypassMux/1 -> emi_125_bypass/1, emi_125/1
  emi_125_bypass/1 -> cfblk148_out1bypassMux/2

== system gm_sampleModel61753_pp_45_1_sub/Subsystem/cfblk150 ==
  emi_132 : Inport  OutDataTypeStr=uint8  PortDimensions=1  SampleTime=1
  Action Port : Inport  Port=2  OutDataTypeStr=boolean  SampleTime=1
  cfblk150 : Subsystem  mask(Real World Value Increment){}
      mask help: Simulink:masks:RealWorldValueIncrement_MD
      mask Display: disp('V++')
  cfblk150_out1bypassMux : MultiPortSwitch  DataPortOrder=Zero-based contiguous  Inputs=2  zeroidx=on  OutDataTypeStr=uint8  SampleTime=1  SaturateOnIntegerOverflow=off  InputSameDT=off
  emi_133_bypass : UnitDelay  InitialCondition="fi(0,0,8,0,\"hex\",\"00\")"  SampleTime=1
  emi_133 : Outport  SampleTime=1  InitialOutput=0
  wires:
  Action Port/1 -> cfblk150_out1bypassMux/1
  emi_132/1 -> cfblk150/1(u)
  cfblk150/1(y) -> cfblk150_out1bypassMux/3
  cfblk150_out1bypassMux/1 -> emi_133_bypass/1, emi_133/1
  emi_133_bypass/1 -> cfblk150_out1bypassMux/2

== system gm_sampleModel61753_pp_45_1_sub/Subsystem/cfblk153 ==
  emi_140 : Inport  OutDataTypeStr=uint8  PortDimensions=1  SampleTime=1
  Action Port : Inport  Port=2  OutDataTypeStr=boolean  SampleTime=1
  cfblk153 : Abs  SampleTime=1  OutDataTypeStr=uint8  SaturateOnIntegerOverflow=off
  cfblk153_out1bypassMux : MultiPortSwitch  DataPortOrder=Zero-based contiguous  Inputs=2  zeroidx=on  OutDataTypeStr=uint8  SampleTime=1  SaturateOnIntegerOverflow=off  InputSameDT=off
  emi_141_bypass : UnitDelay  InitialCondition="fi(0,0,8,0,\"hex\",\"00\")"  SampleTime=1
  emi_141 : Outport  SampleTime=1  InitialOutput=0
  wires:
  Action Port/1 -> cfblk153_out1bypassMux/1
  emi_140/1 -> cfblk153/1
  cfblk153/1 -> cfblk153_out1bypassMux/3
  cfblk153_out1bypassMux/1 -> emi_141_bypass/1, emi_141/1
  emi_141_bypass/1 -> cfblk153_out1bypassMux/2

== system gm_sampleModel61753_pp_45_1_sub/Subsystem/cfblk158 ==
  In1 : Inport  OutDataTypeStr=uint8  PortDimensions=1  SampleTime=1
  Out1 : Outport  SampleTime=1  InitialOutput=[0]
  wires:
  In1/1 -> Out1/1

== system gm_sampleModel61753_pp_45_1_sub/Subsystem/cfblk159 ==
  emi_156 : Inport  OutDataTypeStr=uint8  PortDimensions=1  SampleTime=1
  Action Port : Inport  Port=2  OutDataTypeStr=boolean  SampleTime=1
  cfblk159 : Subsystem
  cfblk159_out1bypassMux : MultiPortSwitch  DataPortOrder=Zero-based contiguous  Inputs=2  zeroidx=on  OutDataTypeStr=uint8  SampleTime=1  SaturateOnIntegerOverflow=off  InputSameDT=off
  emi_157_bypass : UnitDelay  InitialCondition="fi(0,0,8,0,\"hex\",\"00\")"  SampleTime=1
  emi_157 : Outport  SampleTime=1  InitialOutput=0
  wires:
  Action Port/1 -> cfblk159_out1bypassMux/1
  emi_156/1 -> cfblk159/1(In1)
  cfblk159/1(Out1) -> cfblk159_out1bypassMux/3
  cfblk159_out1bypassMux/1 -> emi_157_bypass/1, emi_157/1
  emi_157_bypass/1 -> cfblk159_out1bypassMux/2

== system gm_sampleModel61753_pp_45_1_sub/Subsystem/cfblk160 ==
  In1 : Inport  OutDataTypeStr=uint8  PortDimensions=1  SampleTime=1
  Out1 : Outport  SampleTime=1  InitialOutput=[0]
  wires:
  In1/1 -> Out1/1

== system gm_sampleModel61753_pp_45_1_sub/Subsystem/cfblk165 ==
  emi_116 : Inport  OutDataTypeStr=uint8  PortDimensions=1  SampleTime=1
  Action Port : Inport  Port=2  OutDataTypeStr=boolean  SampleTime=1
  cfblk165 : Subsystem
      settings: MinAlgLoopOccurrences=on
  emi_117 : Outport  SampleTime=1  InitialOutput=0
  wires:
  Action Port/1 -> cfblk165/Enable
  emi_116/1 -> cfblk165/1(in0)
  cfblk165/1(out0) -> emi_117/1

== system gm_sampleModel61753_pp_45_1_sub/Subsystem/cfblk167 ==
  emi_58 : Inport  OutDataTypeStr=uint8  PortDimensions=1  SampleTime=1
  Action Port : Inport  Port=2  OutDataTypeStr=boolean  SampleTime=1
  cfblk167 : Subsystem
      settings: MinAlgLoopOccurrences=on
  emi_59 : Outport  SampleTime=1  InitialOutput=0
  wires:
  Action Port/1 -> cfblk167/Enable
  emi_58/1 -> cfblk167/1(in0)
  cfblk167/1(out0) -> emi_59/1

== system gm_sampleModel61753_pp_45_1_sub/Subsystem/cfblk172 ==
  emi_66 : Inport  OutDataTypeStr=uint8  PortDimensions=1  SampleTime=1
  Action Port : Inport  Port=2  OutDataTypeStr=boolean  SampleTime=1
  cfblk172 : Subsystem
      settings: MinAlgLoopOccurrences=on
  emi_67 : Outport  SampleTime=1  InitialOutput=0
  wires:
  Action Port/1 -> cfblk172/Enable
  emi_66/1 -> cfblk172/1(in0)
  cfblk172/1(out0) -> emi_67/1

== system gm_sampleModel61753_pp_45_1_sub/Subsystem/cfblk180 ==
  emi_148 : Inport  OutDataTypeStr=uint8  PortDimensions=1  SampleTime=1
  Action Port : Inport  Port=2  OutDataTypeStr=boolean  SampleTime=1
  cfblk180 : DataTypeConversion  OutDataTypeStr=fixdt(0,8,0)
  cfblk180_out1bypassMux : MultiPortSwitch  DataPortOrder=Zero-based contiguous  Inputs=2  zeroidx=on  OutDataTypeStr=uint8  SampleTime=1  SaturateOnIntegerOverflow=off  InputSameDT=off
  emi_149_bypass : UnitDelay  InitialCondition="fi(0,0,8,0,\"hex\",\"00\")"  SampleTime=1
  emi_149 : Outport  SampleTime=1  InitialOutput=0
  wires:
  Action Port/1 -> cfblk180_out1bypassMux/1
  emi_148/1 -> cfblk180/1
  cfblk180/1 -> cfblk180_out1bypassMux/3
  cfblk180_out1bypassMux/1 -> emi_149_bypass/1, emi_149/1
  emi_149_bypass/1 -> cfblk180_out1bypassMux/2

== system gm_sampleModel61753_pp_45_1_sub/Subsystem/cfblk19 ==
  emi_164 : Inport  OutDataTypeStr=uint8  PortDimensions=1  SampleTime=1
  Action Port : Inport  Port=2  OutDataTypeStr=boolean  SampleTime=1
  cfblk19 : Abs  SampleTime=1  OutDataTypeStr=uint8  SaturateOnIntegerOverflow=off
  cfblk19_out1bypassMux : MultiPortSwitch  DataPortOrder=Zero-based contiguous  Inputs=2  zeroidx=on  OutDataTypeStr=uint8  SampleTime=1  SaturateOnIntegerOverflow=off  InputSameDT=off
  emi_165_bypass : UnitDelay  InitialCondition="fi(0,0,8,0,\"hex\",\"00\")"  SampleTime=1
  emi_165 : Outport  SampleTime=1  InitialOutput=0
  wires:
  Action Port/1 -> cfblk19_out1bypassMux/1
  emi_164/1 -> cfblk19/1
  cfblk19/1 -> cfblk19_out1bypassMux/3
  cfblk19_out1bypassMux/1 -> emi_165_bypass/1, emi_165/1
  emi_165_bypass/1 -> cfblk19_out1bypassMux/2

== system gm_sampleModel61753_pp_45_1_sub/Subsystem/cfblk192 ==
  emi_180 : Inport  OutDataTypeStr=uint8  PortDimensions=1  SampleTime=1
  Action Port : Inport  Port=2  OutDataTypeStr=boolean  SampleTime=1
  cfblk192 : DataTypeConversion  OutDataTypeStr=fixdt(0,8,0)
  cfblk192_out1bypassMux : MultiPortSwitch  DataPortOrder=Zero-based contiguous  Inputs=2  zeroidx=on  OutDataTypeStr=uint8  SampleTime=1  SaturateOnIntegerOverflow=off  InputSameDT=off
  emi_181_bypass : UnitDelay  InitialCondition="fi(0,0,8,0,\"hex\",\"00\")"  SampleTime=1
  emi_181 : Outport  SampleTime=1  InitialOutput=0
  wires:
  Action Port/1 -> cfblk192_out1bypassMux/1
  emi_180/1 -> cfblk192/1
  cfblk192/1 -> cfblk192_out1bypassMux/3
  cfblk192_out1bypassMux/1 -> emi_181_bypass/1, emi_181/1
  emi_181_bypass/1 -> cfblk192_out1bypassMux/2

== system gm_sampleModel61753_pp_45_1_sub/Subsystem/cfblk194 ==
  emi_188 : Inport  OutDataTypeStr=uint8  PortDimensions=1  SampleTime=1
  Action Port : Inport  Port=2  OutDataTypeStr=boolean  SampleTime=1
  cfblk194 : DataTypeConversion  OutDataTypeStr=fixdt(0,8,0)
  cfblk194_out1bypassMux : MultiPortSwitch  DataPortOrder=Zero-based contiguous  Inputs=2  zeroidx=on  OutDataTypeStr=uint8  SampleTime=1  SaturateOnIntegerOverflow=off  InputSameDT=off
  emi_189_bypass : UnitDelay  InitialCondition="fi(0,0,8,0,\"hex\",\"00\")"  SampleTime=1
  emi_189 : Outport  SampleTime=1  InitialOutput=0
  wires:
  Action Port/1 -> cfblk194_out1bypassMux/1
  emi_188/1 -> cfblk194/1
  cfblk194/1 -> cfblk194_out1bypassMux/3
  cfblk194_out1bypassMux/1 -> emi_189_bypass/1, emi_189/1
  emi_189_bypass/1 -> cfblk194_out1bypassMux/2

== system gm_sampleModel61753_pp_45_1_sub/Subsystem/cfblk2 ==
  note: U(k)
  note: Edge
  U : Inport  OutDataTypeStr=uint8  SampleTime=1
  Delay Input1 : UnitDelay  Description=Store in Global RAM  DisableCoverage=on  InitialCondition=vinit  SampleTime=-1  HasFrameUpgradeWarning=on
  FixPt Relational Operator : RelationalOperator  Operator=>  OutDataTypeStr=fixdt(0, 8)  ZeroCross=off  InputSameDT=off
  Positive : Subsystem  mask(Compare To Zero){relop=>, OutDataTypeStr=boolean, ZeroCross=off}
      mask prompts: relop "Simulink:masks:Operator_MP"; OutDataTypeStr "Simulink:masks:OutputDataType_MP"; ZeroCross "Simulink:masks:EnableZerocrossingDetection_MP"
      mask help: Simulink:masks:CompareToZero_MD
      mask init:
      | OutDataTypeStr = 'boolean';
      | ZeroCross = 'off';
      | blkName = 'sampleModel61753_pp_45_1_sub/Subsystem/cfblk2/Positive';
      | relop = '>';
      | setValue = 'boolean';
      mask TypeOptions relop: == | ~= | < | <= | >= | >
      mask TypeOptions OutDataTypeStr: Simulink:masks:uint8 | Simulink:masks:boolean
      mask Callback ZeroCross: sl('zeroCrossEnable', gcbh);
      mask Display: disp([relop,' 0'])
  Y : Outport  SampleTime=1
  wires:
  U/1 -> Positive/1(u)
  Delay Input1/1 -> FixPt Relational Operator/2
  FixPt Relational Operator/1 -> Y/1
  Positive/1(y) -> FixPt Relational Operator/1, Delay Input1/1

== system gm_sampleModel61753_pp_45_1_sub/Subsystem/cfblk20 ==
  u : Inport  OutDataTypeStr=uint8  SampleTime=1
  FixPt Constant : Constant  DisableCoverage=on  OutDataTypeStr=Inherit: Inherit via back propagation  SampleTime=-1
  FixPt Data Type Duplicate : DataTypeDuplicate  DisableCoverage=on  NumInputPorts=3
  FixPt Sum1 : Sum  OutDataTypeStr=Inherit: Inherit via back propagation  InputSameDT=on  LockScale=on
  y : Outport  SampleTime=1
  wires:
  u/1 -> FixPt Sum1/1, FixPt Data Type Duplicate/2
  FixPt Constant/1 -> FixPt Sum1/2, FixPt Data Type Duplicate/3
  FixPt Sum1/1 -> FixPt Data Type Duplicate/1, y/1

== system gm_sampleModel61753_pp_45_1_sub/Subsystem/cfblk21 ==
  emi_204 : Inport  OutDataTypeStr=uint8  PortDimensions=1  SampleTime=1
  Action Port : Inport  Port=2  OutDataTypeStr=boolean  SampleTime=1
  cfblk21 : Abs  SampleTime=1  OutDataTypeStr=uint8  SaturateOnIntegerOverflow=off
  cfblk21_out1bypassMux : MultiPortSwitch  DataPortOrder=Zero-based contiguous  Inputs=2  zeroidx=on  OutDataTypeStr=uint8  SampleTime=1  SaturateOnIntegerOverflow=off  InputSameDT=off
  emi_205_bypass : UnitDelay  InitialCondition="fi(0,0,8,0,\"hex\",\"00\")"  SampleTime=1
  emi_205 : Outport  SampleTime=1  InitialOutput=0
  wires:
  Action Port/1 -> cfblk21_out1bypassMux/1
  emi_204/1 -> cfblk21/1
  cfblk21/1 -> cfblk21_out1bypassMux/3
  cfblk21_out1bypassMux/1 -> emi_205_bypass/1, emi_205/1
  emi_205_bypass/1 -> cfblk21_out1bypassMux/2

== system gm_sampleModel61753_pp_45_1_sub/Subsystem/cfblk24 ==
  emi_212 : Inport  OutDataTypeStr=uint8  PortDimensions=1  SampleTime=1
  Action Port : Inport  Port=2  OutDataTypeStr=boolean  SampleTime=1
  cfblk24 : Abs  SampleTime=1  OutDataTypeStr=uint8  SaturateOnIntegerOverflow=off
  cfblk24_out1bypassMux : MultiPortSwitch  DataPortOrder=Zero-based contiguous  Inputs=2  zeroidx=on  OutDataTypeStr=uint8  SampleTime=1  SaturateOnIntegerOverflow=off  InputSameDT=off
  emi_213_bypass : UnitDelay  InitialCondition="fi(0,0,8,0,\"hex\",\"00\")"  SampleTime=1
  emi_213 : Outport  SampleTime=1  InitialOutput=0
  wires:
  Action Port/1 -> cfblk24_out1bypassMux/1
  emi_212/1 -> cfblk24/1
  cfblk24/1 -> cfblk24_out1bypassMux/3
  cfblk24_out1bypassMux/1 -> emi_213_bypass/1, emi_213/1
  emi_213_bypass/1 -> cfblk24_out1bypassMux/2

== system gm_sampleModel61753_pp_45_1_sub/Subsystem/cfblk3 ==
  note: U(k)
  note: Edge
  U : Inport  OutDataTypeStr=uint8  SampleTime=1
  Delay Input1 : UnitDelay  Description=Store in Global RAM  DisableCoverage=on  InitialCondition=vinit  SampleTime=-1  HasFrameUpgradeWarning=on
  FixPt Relational Operator : RelationalOperator  Operator=>  OutDataTypeStr=fixdt(0, 8)  ZeroCross=off  InputSameDT=off
  Nonnegative : Subsystem  mask(Compare To Zero){relop=>=, OutDataTypeStr=boolean, ZeroCross=off}
      mask prompts: relop "Simulink:masks:Operator_MP"; OutDataTypeStr "Simulink:masks:OutputDataType_MP"; ZeroCross "Simulink:masks:EnableZerocrossingDetection_MP"
      mask help: Simulink:masks:CompareToZero_MD
      mask init:
      | OutDataTypeStr = 'boolean';
      | ZeroCross = 'off';
      | blkName = 'sampleModel61753_pp_45_1_sub/Subsystem/cfblk3/Nonnegative';
      | relop = '>=';
      | setValue = 'boolean';
      mask TypeOptions relop: == | ~= | < | <= | >= | >
      mask TypeOptions OutDataTypeStr: Simulink:masks:uint8 | Simulink:masks:boolean
      mask Callback ZeroCross: sl('zeroCrossEnable', gcbh);
      mask Display: disp([relop,' 0'])
  Y : Outport  SampleTime=1
  wires:
  U/1 -> Nonnegative/1(u)
  Delay Input1/1 -> FixPt Relational Operator/2
  FixPt Relational Operator/1 -> Y/1
  Nonnegative/1(y) -> FixPt Relational Operator/1, Delay Input1/1

== system gm_sampleModel61753_pp_45_1_sub/Subsystem/cfblk30 ==
  emi_228 : Inport  OutDataTypeStr=uint8  PortDimensions=1  SampleTime=1
  Action Port : Inport  Port=2  OutDataTypeStr=boolean  SampleTime=1
  cfblk30 : Subsystem  mask(Real World Value Increment){}
      mask help: Simulink:masks:RealWorldValueIncrement_MD
      mask Display: disp('V++')
  cfblk30_out1bypassMux : MultiPortSwitch  DataPortOrder=Zero-based contiguous  Inputs=2  zeroidx=on  OutDataTypeStr=uint8  SampleTime=1  SaturateOnIntegerOverflow=off  InputSameDT=off
  emi_229_bypass : UnitDelay  InitialCondition="fi(0,0,8,0,\"hex\",\"00\")"  SampleTime=1
  emi_229 : Outport  SampleTime=1  InitialOutput=0
  wires:
  Action Port/1 -> cfblk30_out1bypassMux/1
  emi_228/1 -> cfblk30/1(u)
  cfblk30/1(y) -> cfblk30_out1bypassMux/3
  cfblk30_out1bypassMux/1 -> emi_229_bypass/1, emi_229/1
  emi_229_bypass/1 -> cfblk30_out1bypassMux/2

== system gm_sampleModel61753_pp_45_1_sub/Subsystem/cfblk31_inst ==
  in1 : Inport  OutDataTypeStr=uint8  SampleTime=1
  in2 : Inport  Port=2  OutDataTypeStr=uint8  SampleTime=1
  mul_cfblk31_dotp_mulcomp : Product  Inputs=**  OutDataTypeStr=uint8  SampleTime=1
  out1 : Outport  OutDataTypeStr=uint8  SampleTime=1
  wires:
  in1/1 -> mul_cfblk31_dotp_mulcomp/1
  in2/1 -> mul_cfblk31_dotp_mulcomp/2
  mul_cfblk31_dotp_mulcomp/1 -> out1/1

== system gm_sampleModel61753_pp_45_1_sub/Subsystem/cfblk33 ==
  u : Inport  OutDataTypeStr=uint8  SampleTime=1
  FixPt Constant : Constant  DisableCoverage=on  OutDataTypeStr=Inherit: Inherit via back propagation  SampleTime=-1
  FixPt Data Type Duplicate : DataTypeDuplicate  DisableCoverage=on  NumInputPorts=3
  FixPt Sum1 : Sum  OutDataTypeStr=Inherit: Inherit via back propagation  InputSameDT=on  LockScale=on
  y : Outport  SampleTime=1
  wires:
  u/1 -> FixPt Sum1/1, FixPt Data Type Duplicate/2
  FixPt Constant/1 -> FixPt Sum1/2, FixPt Data Type Duplicate/3
  FixPt Sum1/1 -> FixPt Data Type Duplicate/1, y/1

== system gm_sampleModel61753_pp_45_1_sub/Subsystem/cfblk37_inst ==
  in1 : Inport  OutDataTypeStr=uint8  SampleTime=1
  in2 : Inport  Port=2  OutDataTypeStr=uint8  SampleTime=1
  mul_cfblk37_dotp_mulcomp : Product  Inputs=**  OutDataTypeStr=uint8  SampleTime=1
  out1 : Outport  OutDataTypeStr=uint8  SampleTime=1
  wires:
  in1/1 -> mul_cfblk37_dotp_mulcomp/1
  in2/1 -> mul_cfblk37_dotp_mulcomp/2
  mul_cfblk37_dotp_mulcomp/1 -> out1/1
